simulink model "das2const"  (Simulink 6.6)
settings: Solver=ode1  StartTime=0.0  StopTime=40  FixedStep=Auto  RelTol=1e-3
settings Model: Creator=chadwick  LastModifiedBy=admin  ParamWorkspaceSource=ReferencedWorkspace  ExtModeAutoUpdateStatusClock=off  BufferReuse=off  ProdHWDeviceType=32-bit xPC Target (Intel Pentium)
settings DataIOCC: MaxDataPoints=20000  SaveFinalState=on  SaveOutput=off  SignalLogging=off  SaveTime=off
settings OptimizationCC: BlockReduction=off  InlineParams=on  OptimizeBlockIOStorage=off  BufferReuse=off  ExpressionFolding=off  LocalBlockOutputs=off
settings DebuggingCC: SignalResolutionControl=TryResolveAllWithWarning  MultiTaskDSMMsg=warning  MultiTaskCondExecSysMsg=none
settings HardwareCC: ProdIntDivRoundTo=Zero  ProdEndianess=LittleEndian  ProdHWDeviceType=32-bit xPC Target (Intel Pentium)
settings ModelReferenceCC: ModelReferenceNumInstancesAllowed=Single
settings RTWCC: SystemTargetFile=xpctarget.tlc  TemplateMakefile=xpc_default_tmf  Description=xPC Target  ProcessScript=xpctarget_make_rtw_hook  CustomInclude=..\..\..\tools\sdbio\trunk\ ..\..\..\das2\model\trunk\ ..\..\..\das2\das2sim\trunk\  CustomSource=sdbio.c sdlib.c model_d.c  IncludeERTFirstTime=on
settings xpcTargetCC: TargetFcnLib=ansi_tfl_tmw.mat  GenFloatMathFcnCalls=ANSI_C  PortableWordSizes=off  RL32ModeModifier=Freerun  RL32LogBufSizeModifier=20000

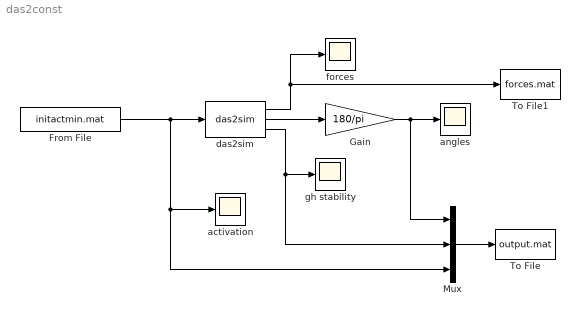
== system das2const ==
  From File : FromFile  FileName=initactmin.mat  SampleTime=0.0004
  Gain : Gain  Gain=180/pi
  Mux : Mux  Inputs=3
  To File : ToFile  Filename=output.mat  MatrixName=output
      settings: Decimation=10
  To File1 : ToFile  Filename=forces.mat  MatrixName=forces
      settings: Decimation=10
  activation : Scope
      settings: YMin=0  YMax=0.07  SaveName=ScopeData2  MaxDataPoints=10000  Decimation=10
  angles : Scope
      settings: YMin=-10  YMax=75  MaxDataPoints=10000  Decimation=10
  das2sim : S-Function  FunctionName=das2sim
  forces : Scope
      settings: YMin=-1  YMax=13  SaveName=ScopeData3  MaxDataPoints=10000  Decimation=10
  gh stability : Scope
      settings: YMin=0  YMax=0.4  MaxDataPoints=10000  Decimation=10
  wires:
  das2sim/2 -> Gain/1
  Gain/1 -> angles/1, Mux/1
  das2sim/3 -> gh stability/1, Mux/2
  Mux/1 -> To File/1
  das2sim/1 -> forces/1, To File1/1
  From File/1 -> das2sim/1, activation/1, Mux/3
